simulink library "uas_pilot_model_r6"  (R2018b)
settings: Solver=VariableStepAuto  StartTime=0.0  StopTime=10.0  RelTol=1e-3
values from neighbouring files (symbols this model uses):
  deterministicMode = false    [HeuristicOperatorModelR6.m]
undefined symbols (not defined in the file or in its folder): alt_k, alt_offset, alt_theta, coord_delay_k, coord_delay_min, coord_delay_theta, dt, max_hdg_diff, mean_exec_delay, mean_initial_delay, mean_upd_times, min_exec_delay, min_initial_delay, min_upd_times, operator_enabled, prob_descend, prob_follow_min, prob_turn, prob_turn_left, rng_seed_coord, rng_seed_execution, rng_seed_horz, rng_seed_horz_vs_vert, rng_seed_initial, rng_seed_update, rng_seed_vert, turn_k, turn_k_alt, turn_offset, turn_offset_alt, turn_theta, turn_theta_alt
libraries: simulink x10
(part 2 of 2)

== matlab function uas_pilot_model_r6/UAS Pilot Model Release 6.1/Use Pilot Model/Maneuver/Maneuver Selection/Draw Vertical Magnitude/MATLAB Function ==
  data: maneuver input; magnitude output; k input; theta input; offset input; seed input
function magnitude = fcn(maneuver, k, theta, offset, seed)
%#codegen

magnitude = HeuristicOperatorModelR6_ExternalFunctions.drawManeuverMagnitude(maneuver, k, theta, offset, seed);

== matlab function uas_pilot_model_r6/UAS Pilot Model Release 6.1/Use Pilot Model/Maneuver/Maneuver Selection/Get Minimum Maneuvers/Get Minimum Altitudes ==
  data: bands input; alts output; wc_flag output; currAlt input
function [alts, wc_flag] = fcn(bands, currAlt)
%#codegen

% pre-define output variable
alts = [0; 0]; %#ok<NASGU>
wc_flag = [0; 0]; %#ok<NASGU>

[alts, wc_flag] = HeuristicOperatorModelR6_ExternalFunctions.getMinimumAltitudes(bands, currAlt);

== matlab function uas_pilot_model_r6/UAS Pilot Model Release 6.1/Use Pilot Model/Maneuver/Maneuver Selection/Get Minimum Maneuvers/Get Minimum Turns ==
  data: bands input; turns output; wc_flag output
function [turns, wc_flag] = fcn(bands)
%#codegen

% pre-define output variable
turns = [0; 0]; %#ok<NASGU>
wc_flag = [0; 0]; %#ok<NASGU>

[turns, wc_flag] = HeuristicOperatorModelR6_ExternalFunctions.getMinimumTurns(bands);

== matlab function uas_pilot_model_r6/UAS Pilot Model Release 6.1/Use Pilot Model/Maneuver/Maneuver Selection/Vertical Maneuver Heuristic/Minimum Maneuver Heuristic ==
  data: maneuvers input; index output; wc_flags input; preference_min input; preference_dir input; seed input
function index = fcn(maneuvers, wc_flags, preference_min, preference_dir, seed)
%#codegen

index = 0;
max_diff = 1e6;
index = HeuristicOperatorModelR6_ExternalFunctions.chooseMinimumManeuver(maneuvers, wc_flags, preference_min, preference_dir, max_diff, seed);
